simulink model "quad_model_with_pendulum"  (R2016a)
settings: Solver=ode45  StartTime=0.0  StopTime=30  RelTol=1e-3
values from neighbouring files (symbols this model uses):
  disturbance_xy_wind_gain = 0.00    (= 0)    [quad_model_with_pendulum_params.m]
  disturbance_y_delay = 0.5    [quad_model_with_pendulum_params.m]
  gravity = 9.80665    [quad_model_with_pendulum_params.m]
  has_links = 1    [quad_model_with_pendulum_params.m]
  has_sensor = 1    [quad_model_with_pendulum_params.m]
  link_length = 0.25    [quad_model_with_pendulum_params.m]
  link_mass = 0.0075/2    (= 0.00375)    [quad_model_with_pendulum_params.m]
  N = 1    [quaternion.m]
  num_links = 16    [quad_model_with_pendulum_params.m]
  s = ones( size( x ))    [quaternion.m]
  sensor_delay = 0.30    (= 0.3)    [quad_model_with_pendulum_params.m]
  sensor_mass = 0.015    [quad_model_with_pendulum_params.m]
  sensor_sample_time = 0.1    [quad_model_with_pendulum_params.m]
  vehicle_initial_height = -4    [quad_model_with_pendulum_params.m]
  vehicle_mass = 0.550    (= 0.55)    [quad_model_with_pendulum_params.m]
  vehicle_velocity_ascent_limit = -4    [quad_model_with_pendulum_params.m]
  vehicle_velocity_descent_limit = 4.0    (= 4)    [quad_model_with_pendulum_params.m]
  w_ref = 0    [quad_model_with_pendulum_params.m]
  x_Kd = 0.14/n    (= 0.14)    [quad_model_with_pendulum_params.m]
  x_Kp = 0.085/n    (= 0.085)    [quad_model_with_pendulum_params.m]
  x_ref = 1    [quad_model_with_pendulum_params.m]
  Y = [Y(1,:); Y(end,:)]    [quaternion.m]
  y_Kd = 0.14/n    (= 0.14)    [quad_model_with_pendulum_params.m]
  y_Kp = 0.085/n    (= 0.085)    [quad_model_with_pendulum_params.m]
  y_ref = 1    [quad_model_with_pendulum_params.m]
  z_Kd = 1.05    [quad_model_with_pendulum_params.m]
  z_Kp = 0.8    [quad_model_with_pendulum_params.m]
  z_ref = 0.0    (= 0)    [quad_model_with_pendulum_params.m]
undefined symbols (not defined in the file or in its folder): EulerAngles, quaternion, RotateVector, wind_velocity_scale_factor, X, Z
libraries: nesl_utility x21, sm_lib x17, experimental_link_model_x_plus x8, experimental_link_model_x_minus x7, dsparch4 x3, simulink x3, fuzblock x2
settings Model: Creator=jore  LastModifiedBy=jore
settings DataIOCC: LimitDataPoints=on  SaveFormat=Array  OutputTimes=[0:0.3:30]
settings HardwareCC: ProdBitPerPointer=32  ProdLargestAtomicFloat=None  ProdIntDivRoundTo=Undefined  ProdEndianess=Unspecified  ProdWordSize=32  ProdHWDeviceType=32-bit Generic
settings ModelReferenceCC: PropagateSignalLabelsOutOfModel=off
settings ConfigComp: CovModelRefEnable=Off
settings ConfigurationSet: Description=SimMechanics 2G
settings ExplorerConfigSet: InternalSimMechanicsExplorerSettings="<ExplorerConfiguration><canonicalview>aerospace</canonicalview><AnimationSetting><BasePlaybackSpeed>1.0</BasePlaybackSpeed><PlaybackSpeedFactor>1.0</PlaybackSpeedFactor></AnimationSetting><TilePanel><TileInfo><Tiles Columns=\"1\" Count=\"1\" Rows=\"1\"><Column Left=\"2\" Weight=\"1\"/><Column Left=\"883\"/><Row Top=\"2\" Weight=\"1\"/><Row Top=\"2319\"/><Tile Height=\"1\" Width=\"1\" X=\"0\" Y=\"0\"/></Tiles></TileInfo><SceneInfo><SceneViewer><BGColor><R>0.60000002384185791</R><G>0.60000002384185791</G><B>0.60000002384185791</B></BGColor><Camera><DoPerspective>off</DoPerspective><Position><X>0.206725447032578502</X><Y>12.9211399937233526</Y><Z>-2.23169927424554082</Z></Position><Center><X>0.206725447032578502</X><Y>-6.73147066983237341e-07</Y><Z>-2.23169927424554082</Z></Center><Up><X>0</X><Y>0</Y><Z>-1</Z></Up><ViewLimDist>1</ViewLimDist><YLim>10.4733537019934797</YLim><XLim>3.95700365170637491</XLim></Camera></SceneViewer></SceneInfo></TilePanel><MechEditorPanel><Cameras/><GfxPanelCameraMap/></MechEditorPanel></ExplorerConfiguration>"

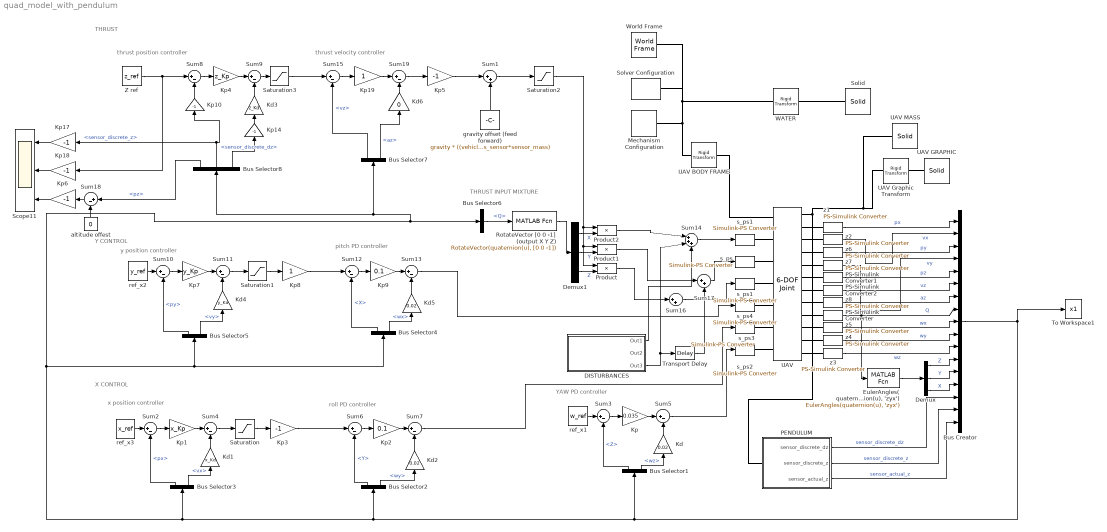
== system quad_model_with_pendulum ==
  note: THRUST INPUT MIXTURE
  note: X CONTROL
  note: THRUST
  note: YAW PD controller
  note: x position controller
  note: roll PD controller
  note: y position controller
  note: pitch PD controller
  note: thrust position controller
  note: thrust velocity controller
  note: Y CONTROL
   s_ps{1..4} (4 alike) : nesl_utility/Simulink-PS Converter  PhysicalDomain=network_engine_domain  SubClassName=ps_input  LeftPortType=input  RightPortType=output  PseudoPeriodic=off  Frequencies=[]  NoiseDistribution=none  NoiseParameters=[]  Unit=1  AffineConversion=off  InputFiltering=off  SimscapeFilterOrder=1  InputFilterTimeConstant=0.001  UdotUserProvided=1
  Bus Creator : BusCreator  Inputs=17
  Bus Selector1 : BusSelector  OutputSignals=Z,wz
  Bus Selector2 : BusSelector  OutputSignals=Y,wy
  Bus Selector3 : BusSelector  OutputSignals=px,vx
  Bus Selector4 : BusSelector  OutputSignals=X,wx
  Bus Selector5 : BusSelector  OutputSignals=py,vy
  Bus Selector6 : BusSelector  OutputSignals=Q
  Bus Selector7 : BusSelector  OutputSignals=vz,az
  Bus Selector8 : BusSelector  OutputSignals=pz,sensor_discrete_z,sensor_discrete_dz
  DISTURBANCES : Subsystem
  Demux : Demux  Outputs=3
  Demux1 : Demux  Outputs=3
  "EulerAngles( quaternion(u), 'zyx')" : MATLABFcn  MATLABFcn=EulerAngles(quaternion(u), 'zyx')  OutputDimensions=3
  Kd : Gain  Gain=0.02
  Kd1 : Gain  Gain=x_Kd
  Kd2 : Gain  Gain=0.02
  Kd3 : Gain  Gain=z_Kd
  Kd4 : Gain  Gain=y_Kd
  Kd5 : Gain  Gain=0.02
  Kd6 : Gain  Gain=0
  Kp : Gain  Gain=0.035
  Kp1 : Gain  Gain=x_Kp
  Kp{3,5..6,10,14,17..18} (7 alike) : Gain  Gain=-1
  Kp19 : Gain
  Kp2 : Gain  Gain=0.1
  Kp4 : Gain  Gain=z_Kp
  Kp7 : Gain  Gain=y_Kp
  Kp8 : Gain
  Kp9 : Gain  Gain=0.1
  Mechanism Configuration : sm_lib/Utilities/Mechanism Configuration  UniformGravity=Constant  GravityVector=[0 0 9.80665]  GravityUnits=m/s^2  LinearizationDelta=0.001
  PENDULUM : Subsystem
  PS-Simulink Converter : nesl_utility/PS-Simulink Converter  PhysicalDomain=network_engine_domain  SubClassName=ps_output  LeftPortType=input  RightPortType=output  PseudoPeriodic=off  Frequencies=[]  Unit=1  AffineConversion=off
  PS-Simulink Converter1 : nesl_utility/PS-Simulink Converter  PhysicalDomain=network_engine_domain  SubClassName=ps_output  LeftPortType=input  RightPortType=output  PseudoPeriodic=off  Frequencies=[]  Unit=1  AffineConversion=off
  PS-Simulink Converter2 : nesl_utility/PS-Simulink Converter  PhysicalDomain=network_engine_domain  SubClassName=ps_output  LeftPortType=input  RightPortType=output  PseudoPeriodic=off  Frequencies=[]  Unit=1  AffineConversion=off
  Product : Product
  Product1 : Product
  Product2 : Product
  RotateVector [0 0 -1] (output X Y Z) : MATLABFcn  MATLABFcn=RotateVector(quaternion(u), [0 0 -1])  OutputDimensions=3
  Saturation : Saturate  UpperLimit=pi/30  LowerLimit=-pi/30
  Saturation1 : Saturate  UpperLimit=pi/30  LowerLimit=-pi/30
  Saturation2 : Saturate  UpperLimit=20  LowerLimit=5.3
  Saturation3 : Saturate  UpperLimit=vehicle_velocity_descent_limit  LowerLimit=vehicle_velocity_ascent_limit
  Scope11 : Scope  NumInputPorts=3
  Solid : sm_lib/Body Elements/Solid  InertiaType=PointMass  Mass=0  MassUnits=kg  CenterOfMass=[0 0 0]  CenterOfMassUnits=m  MomentsOfInertia=[1 1 1]  MomentsOfInertiaUnits=kg*m^2  ProductsOfInertia=[0 0 0]  ProductsOfInertiaUnits=kg*m^2  DensityBased=on  Density=1000  DensityUnits=kg/(m^3)  DoExposeReferenceFrame=on  SerializedFrames=<Frames/>  GraphicType=FromGeometry  MarkerShape=Sphere  MarkerSize=10  MarkerSizeUnits=m  GraphicVisPropType=SimpleVisualProperties  GraphicDiffuseColor=[0.2 0.6 1.0]  GraphicSpecularColor=[0.5 0.5 0.5 1.0]  GraphicAmbientColor=[0.15 0.15 0.15 1.0]  GraphicEmissiveColor=[0.0 0.0 0.0 1.0]  GraphicShininess=75  GraphicOpacity=0.3  GeometryShape=Cylinder  RectangleSize=[1 1]  RectangleSizeUnits=m  BrickDimensions=[1 1 1]  BrickDimensionUnits=m  CylinderRadius=9  CylinderRadiusUnits=m  CylinderLength=4  CylinderLengthUnits=m  SphereRadius=1  SphereRadiusUnits=m  EllipsoidRadii=[1 1 1]  EllipsoidRadiiUnits=m  ExtrusionCrossSection=[1 1; -1 1; -1 -1; 1 -1]  ExtrusionCrossSectionUnits=m  ExtrusionLength=1  ExtrusionLengthUnits=m  PolygonNumSides=3  PolygonOuterRadius=1  PolygonOuterRadiusUnits=m  ExtGeomFileType=STL  ExtGeomFileUnits=m  RevolutionCrossSection=[1 1; 1 -1; 2 -1; 2 1]  RevolutionCrossSectionUnits=m  RevolutionExtent=Full  RevolutionAngle=180  RevolutionAngleUnits=deg
  Solver Configuration : nesl_utility/Solver Configuration  PhysicalDomain=network_engine_domain  SubClassName=solver  LeftPortType=input  RightPortType=generic  Accelerate=off  Tones=[]  Harmonics=[]  SimulateNoise=off  Profile=off  UseLocalSampling=off  EnableSwitchedLinearOptims=on  FrequencyDomain=off  UseCCode=off  RelTol=0.001  AbsTol=1e-06  MinStep=1e-09  ToWorkspace=off  RevertToSquareIcSolve=off  NumHomotopyIterations=100  PhasorMode=off  PhasorModeNumHarmonics=1  OverrideAbsTol=off  DoDC=off  ResidualTolerance=1e-09  UseLocalSolver=off  LocalSolverChoice=NE_BACKWARD_EULER_ADVANCER  LocalSolverSampleTime=0.0001  DoFixedCost=off  MaxNonlinIter=3  MaxModeIter=2  LinearAlgebra=Sparse  DelaysMemoryBudget=1024  AutomaticFiltering=on  FilteringTimeConstant=0.001
  Sum1 : Sum  Inputs=|++
  Sum{2..13,15,18..19} (15 alike) : Sum  Inputs=|+-
  Sum14 : Sum  Inputs=|+++
  Sum16 : Sum  Inputs=|++
  Sum17 : Sum  Inputs=|++
  To Workspace1 : ToWorkspace  VariableName=x1  SaveFormat=Timeseries  SampleTime=-1
  Transport Delay : TransportDelay  DelayTime=disturbance_y_delay
  UAV : sm_lib/Joints/6-DOF Joint  SenseConstraintForce=off  SenseConstraintForceX=off  SenseConstraintForceY=off  SenseConstraintForceZ=off  SenseConstraintTorque=off  SenseConstraintTorqueX=off  SenseConstraintTorqueY=off  SenseConstraintTorqueZ=off  SenseTotalForce=off  SenseTotalForceX=off  SenseTotalForceY=off  SenseTotalForceZ=off  SenseTotalTorque=off  SenseTotalTorqueX=off  SenseTotalTorqueY=off  SenseTotalTorqueZ=off  CompositeWrenchDir=FollowerOnBase  CompositeWrenchFrame=BaseFrame  PxEquilibriumPosition=0  PxEquilibriumPositionUnits=m  PxSpringStiffness=0  PxSpringStiffnessUnits=N/m  PxDampingCoefficient=0  PxDampingCoefficientUnits=N/(m/s)  PxTorqueActuationMode=InputTorque  PxMotionActuationMode=ComputedMotion  PxSensePosition=on  PxSenseVelocity=on  PxSenseAcceleration=off  PxSenseTorqueForce=off  PxPositionTargetSpecify=off  PxPositionTargetPriority=High  PxPositionTargetValue=0  PxPositionTargetValueUnits=m  PxVelocityTargetSpecify=off  PxVelocityTargetPriority=High  PxVelocityTargetValue=0  PxVelocityTargetValueUnits=m/s  PyEquilibriumPosition=0  PyEquilibriumPositionUnits=m  PySpringStiffness=0  PySpringStiffnessUnits=N/m  PyDampingCoefficient=0  PyDampingCoefficientUnits=N/(m/s)  PyTorqueActuationMode=InputTorque  PyMotionActuationMode=ComputedMotion  PySensePosition=on  PySenseVelocity=on  PySenseAcceleration=off  PySenseTorqueForce=off  PyPositionTargetSpecify=off  PyPositionTargetPriority=High  PyPositionTargetValue=0  PyPositionTargetValueUnits=m  PyVelocityTargetSpecify=off  PyVelocityTargetPriority=High  PyVelocityTargetValue=0  PyVelocityTargetValueUnits=m/s  PzEquilibriumPosition=0  PzEquilibriumPositionUnits=m  PzSpringStiffness=0  PzSpringStiffnessUnits=N/m  PzDampingCoefficient=0  PzDampingCoefficientUnits=N/(m/s)  PzTorqueActuationMode=InputTorque  PzMotionActuationMode=ComputedMotion  PzSensePosition=on  PzSenseVelocity=on  PzSenseAcceleration=on  PzSenseTorqueForce=off  PzPositionTargetSpecify=on  PzPositionTargetPriority=High  PzPositionTargetValue=0  PzPositionTargetValueUnits=m  PzVelocityTargetSpecify=off  PzVelocityTargetPriority=High  PzVelocityTargetValue=0  PzVelocityTargetValueUnits=m/s  SphDefPosRotationMethod=None  SphDefPosRotationAngleUnits=deg  SphDefPosRotationStandardAxis=+Z  SphDefPosRotationAngle=0.0  SphDefPosRotationArbitraryAxis=[0 0 1]  SphDefPosFollAlignAxisA=+X  SphDefPosBaseAlignAxisA=+Y  SphDefPosFollAlignAxisB=+Y  SphDefPosBaseAlignAxisB=+Z  SphDefPosRotationSequenceAxes=FollowerAxes  SphDefPosRotationSequence=XYX  SphDefPosRotationSequenceAngles=[0 0 0]  SphDefPosRotationSequenceAnglesUnits=deg  SphDefPosRotationMatrix=[1 0 0; 0 1 0; 0 0 1]  SphEqPosRotationMethod=None  SphEqPosRotationAngleUnits=deg  SphEqPosRotationStandardAxis=+Z  SphEqPosRotationAngle=0.0  SphEqPosRotationArbitraryAxis=[0 0 1]  SphEqPosFollAlignAxisA=+X  SphEqPosBaseAlignAxisA=+Y  SphEqPosFollAlignAxisB=+Y  SphEqPosBaseAlignAxisB=+Z  SphEqPosRotationSequenceAxes=FollowerAxes  SphEqPosRotationSequence=XYX  SphEqPosRotationSequenceAngles=[0 0 0]  SphEqPosRotationSequenceAnglesUnits=deg  SphEqPosRotationMatrix=[1 0 0; 0 1 0; 0 0 1]  SphSpringStiffness=0  SphSpringStiffnessUnits=N*m/deg  SphDampingCoefficient=0  SphDampingCoefficientUnits=N*m/(deg/s)  SphActuateTorqueX=on  SphActuateTorqueY=on  SphActuateTorqueZ=on  SphActuateTorque=off  SphTorqueActuationMode=InputTorque  SphMotionActuationMode=ComputedMotion  SphActuationFrame=BaseFrame  SphSensePosition=on  SphSenseVelocityX=on  SphSenseVelocityY=on  SphSenseVelocityZ=on  SphSenseVelocity=off  SphSenseAccelerationX=off  SphSenseAccelerationY=off  SphSenseAccelerationZ=off  SphSenseAcceleration=off  SphSenseTorqueX=off  SphSenseTorqueY=off  SphSenseTorqueZ=off  SphSenseTorqueForce=off  SphSensingFrame=BaseFrame  SphPositionTargetRotationMethod=None  SphPositionTargetRotationAngleUnits=deg  SphPositionTargetRotationStandardAxis=+Z  SphPositionTargetRotationAngle=0.0  SphPositionTargetRotationArbitraryAxis=[0 0 1]  SphPositionTargetFollAlignAxisA=+X  SphPositionTargetBaseAlignAxisA=+Y  SphPositionTargetFollAlignAxisB=+Y  SphPositionTargetBaseAlignAxisB=+Z  SphPositionTargetRotationSequenceAxes=FollowerAxes  SphPositionTargetRotationSequence=XYX  SphPositionTargetRotationSequenceAngles=[0 0 0]  SphPositionTargetRotationSequenceAnglesUnits=deg  SphPositionTargetRotationMatrix=[1 0 0; 0 1 0; 0 0 1]  SphPositionTargetSpecify=off  SphPositionTargetPriority=High  SphVelocityTargetValue=[0 0 0]  SphVelocityTargetValueUnits=deg/s  SphVelocityTargetSpecify=off  SphVelocityTargetPriority=High  SphVelocityTargetInFollowerFrame=on
  UAV BODY FRAME : sm_lib/Frames and Transforms/Rigid Transform  TranslationMethod=Cartesian  TranslationLengthUnit=m  TranslationStandardAxis=-Z  TranslationStandardOffset=num_links*link_length  TranslationCartesianOffset="[0 0  vehicle_initial_height]"  TranslationROffset=0  TranslationROffsetUnits=m  TranslationZOffset=0  TranslationZOffsetUnits=m  TranslationThetaOffset=0  TranslationThetaOffsetUnits=deg  RotationMethod=None  RotationAngleUnits=deg  RotationStandardAxis=+X  RotationAngle=90  RotationArbitraryAxis=[0 1 1]  FollAlignAxisA=+X  BaseAlignAxisA=+Y  FollAlignAxisB=+Y  BaseAlignAxisB=+Z  RotationSequenceAxes=FollowerAxes  RotationSequence=XYX  RotationSequenceAngles=[0 0 0]  RotationSequenceAnglesUnits=deg  RotationMatrix=[0 0 1; -1 0 0; 0 -1 0]
  UAV GRAPHIC : sm_lib/Body Elements/Solid  InertiaType=PointMass  Mass=0  MassUnits=kg  CenterOfMass=[0 0 0]  CenterOfMassUnits=m  MomentsOfInertia=[1 1 1]  MomentsOfInertiaUnits=kg*m^2  ProductsOfInertia=[0 0 0]  ProductsOfInertiaUnits=kg*m^2  DensityBased=off  Density=1000  DensityUnits=kg/(m^3)  DoExposeReferenceFrame=on  SerializedFrames=<Frames/>  GraphicType=FromGeometry  MarkerShape=Sphere  MarkerSize=10  MarkerSizeUnits=m  GraphicVisPropType=SimpleVisualProperties  GraphicDiffuseColor=[0.3 0.3 0.3]  GraphicSpecularColor=[0.5 0.5 0.5 1.0]  GraphicAmbientColor=[0.15 0.15 0.15 1.0]  GraphicEmissiveColor=[0.0 0.0 0.0 1.0]  GraphicShininess=75  GraphicOpacity=1.0  GeometryShape=FromFile  RectangleSize=[1 1]  RectangleSizeUnits=m  BrickDimensions=[1 1 1]  BrickDimensionUnits=m  CylinderRadius=1  CylinderRadiusUnits=m  CylinderLength=1  CylinderLengthUnits=m  SphereRadius=1  SphereRadiusUnits=m  EllipsoidRadii=[1 1 1]  EllipsoidRadiiUnits=m  ExtrusionCrossSection=[1 1; -1 1; -1 -1; 1 -1]  ExtrusionCrossSectionUnits=m  ExtrusionLength=1  ExtrusionLengthUnits=m  PolygonNumSides=3  PolygonOuterRadius=1  PolygonOuterRadiusUnits=m  ExtGeomFileType=STL  ExtGeomFileName=Top Level Hummingbird Part.STL  ExtGeomFileUnits=mm  RevolutionCrossSection=[1 1; 1 -1; 2 -1; 2 1]  RevolutionCrossSectionUnits=m  RevolutionExtent=Full  RevolutionAngle=180  RevolutionAngleUnits=deg
  UAV Graphic Transform : sm_lib/Frames and Transforms/Rigid Transform  TranslationMethod=Cartesian  TranslationLengthUnit=m  TranslationStandardAxis=+Z  TranslationStandardOffset=0  TranslationCartesianOffset=[-0.275 0.238 0.02]  TranslationROffset=0  TranslationROffsetUnits=m  TranslationZOffset=0  TranslationZOffsetUnits=m  TranslationThetaOffset=0  TranslationThetaOffsetUnits=deg  RotationMethod=RotationMatrix  RotationAngleUnits=deg  RotationStandardAxis=+X  RotationAngle=90  RotationArbitraryAxis=[0 1 1]  FollAlignAxisA=+X  BaseAlignAxisA=+Y  FollAlignAxisB=+Y  BaseAlignAxisB=+Z  RotationSequenceAxes=FollowerAxes  RotationSequence=XYX  RotationSequenceAngles=[0 0 0]  RotationSequenceAnglesUnits=deg  RotationMatrix=[0 0 1; -1 0 0; 0 -1 0]
  UAV MASS : sm_lib/Body Elements/Solid  InertiaType=CalculateFromGeometry  Mass=vehicle_mass  MassUnits=kg  CenterOfMass=[0 0 0]  CenterOfMassUnits=m  MomentsOfInertia=[1 1 1]  MomentsOfInertiaUnits=kg*m^2  ProductsOfInertia=[0 0 0]  ProductsOfInertiaUnits=kg*m^2  DensityBased=off  Density=1  DensityUnits=kg/(m^3)  DoExposeReferenceFrame=on  SerializedFrames=<Frames/>  GraphicType=None  MarkerShape=Sphere  MarkerSize=10  MarkerSizeUnits=m  GraphicVisPropType=SimpleVisualProperties  GraphicDiffuseColor=[1.0 1.0 0.2]  GraphicSpecularColor=[0.5 0.5 0.5 1.0]  GraphicAmbientColor=[0.15 0.15 0.15 1.0]  GraphicEmissiveColor=[0.0 0.0 0.0 1.0]  GraphicShininess=75  GraphicOpacity=0.1  GeometryShape=Sphere  RectangleSize=[1 1]  RectangleSizeUnits=m  BrickDimensions=[1 1 1]  BrickDimensionUnits=m  CylinderRadius=1  CylinderRadiusUnits=m  CylinderLength=1  CylinderLengthUnits=m  SphereRadius=0.1  SphereRadiusUnits=m  EllipsoidRadii=[1 1 1]  EllipsoidRadiiUnits=m  ExtrusionCrossSection=[1 1; -1 1; -1 -1; 1 -1]  ExtrusionCrossSectionUnits=m  ExtrusionLength=1  ExtrusionLengthUnits=m  PolygonNumSides=3  PolygonOuterRadius=1  PolygonOuterRadiusUnits=m  ExtGeomFileType=STL  ExtGeomFileUnits=m  RevolutionCrossSection=[1 1; 1 -1; 2 -1; 2 1]  RevolutionCrossSectionUnits=m  RevolutionExtent=Full  RevolutionAngle=180  RevolutionAngleUnits=deg
  WATER : sm_lib/Frames and Transforms/Rigid Transform  TranslationMethod=StandardAxis  TranslationLengthUnit=m  TranslationStandardAxis=+Z  TranslationStandardOffset=2  TranslationCartesianOffset=[-0.275 0.238 0.02]  TranslationROffset=0  TranslationROffsetUnits=m  TranslationZOffset=0  TranslationZOffsetUnits=m  TranslationThetaOffset=0  TranslationThetaOffsetUnits=deg  RotationMethod=None  RotationAngleUnits=deg  RotationStandardAxis=+X  RotationAngle=90  RotationArbitraryAxis=[0 1 1]  FollAlignAxisA=+X  BaseAlignAxisA=+Y  FollAlignAxisB=+Y  BaseAlignAxisB=+Z  RotationSequenceAxes=FollowerAxes  RotationSequence=XYX  RotationSequenceAngles=[0 0 0]  RotationSequenceAnglesUnits=deg  RotationMatrix=[0 0 1; -1 0 0; 0 -1 0]
  World Frame : sm_lib/Frames and Transforms/World Frame
  "Z ref " : Constant  Value=z_ref
  altitude offest : Constant  Value=0
  gravity offset (feed forward) : Constant  Value=gravity * ((vehicle_mass) + has_links*(num_links * link_mass) + has_sensor*sensor_mass)
  ref_x1 : Constant  Value=w_ref
  ref_x2 : Constant  Value=y_ref
  ref_x3 : Constant  Value=x_ref
  s_ps : nesl_utility/Simulink-PS Converter  PhysicalDomain=network_engine_domain  SubClassName=ps_input  LeftPortType=input  RightPortType=output  PseudoPeriodic=off  Frequencies=[]  NoiseDistribution=none  NoiseParameters=[]  Unit=1  AffineConversion=off  InputFiltering=off  SimscapeFilterOrder=1  InputFilterTimeConstant=0.001  UdotUserProvided=1
  s_ps1 : nesl_utility/Simulink-PS Converter  PhysicalDomain=network_engine_domain  SubClassName=ps_input  LeftPortType=input  RightPortType=output  PseudoPeriodic=off  Frequencies=[]  NoiseDistribution=none  NoiseParameters=[]  Unit=1  AffineConversion=off  InputFiltering=off  SimscapeFilterOrder=1  InputFilterTimeConstant=0.001  UdotUserProvided=1
  z{1..8} (8 alike) : nesl_utility/PS-Simulink Converter  PhysicalDomain=network_engine_domain  SubClassName=ps_output  LeftPortType=input  RightPortType=output  PseudoPeriodic=off  Frequencies=[]  Unit=1  AffineConversion=off
  wires:
  PS-Simulink Converter/1 -> Bus Creator/8, "EulerAngles( quaternion(u), 'zyx')"/1  "Q"
  "EulerAngles( quaternion(u), 'zyx')"/1 -> Demux/1
  Demux/1 -> Bus Creator/12  "Z"
  Kd/1 -> Sum5/2
  z3/1 -> Bus Creator/11  "wz"
  Sum3/1 -> Kp/1
  Kp/1 -> Sum5/1
  ref_x1/1 -> Sum3/1
  RotateVector [0 0 -1] (output X Y Z)/1 -> Demux1/1
  Demux1/3 -> Product/2  "Z"
  gravity offset (feed forward)/1 -> Sum1/2
  Demux1/1 -> Product2/2  "X"
  Demux1/2 -> Product1/2  "Y"
  Sum5/1 -> " s_ps2"/1
  Sum2/1 -> Kp1/1
  Kp1/1 -> Sum4/1
  ref_x3/1 -> Sum2/1
  z1/1 -> Bus Creator/1  "px"
  Product2/1 -> Sum14/1
  Product/1 -> Sum16/1
  Kd2/1 -> Sum7/2
  Sum6/1 -> Kp2/1
  Kp2/1 -> Sum7/1
  Demux/2 -> Bus Creator/13  "Y"
  z4/1 -> Bus Creator/10  "wy"
  Sum4/1 -> Saturation/1
  Sum7/1 -> " s_ps3"/1
  Saturation/1 -> Kp3/1
  Kp3/1 -> Sum6/1
  Kd1/1 -> Sum4/2
  z2/1 -> Bus Creator/2  "vx"
  Sum8/1 -> Kp4/1
  Kp4/1 -> Sum9/1
  "Z ref "/1 -> Kp18/1, Sum8/1
  PS-Simulink Converter1/1 -> Bus Creator/5  "pz"
  PS-Simulink Converter2/1 -> Bus Creator/6  "vz"
  Kp5/1 -> Sum1/1
  Kd3/1 -> Sum9/2
  Kp6/1 -> Scope11/3
  Sum10/1 -> Kp7/1
  Kp7/1 -> Sum11/1
  ref_x2/1 -> Sum10/1
  Sum11/1 -> Saturation1/1
  Saturation1/1 -> Kp8/1
  Kd4/1 -> Sum11/2
  Kd5/1 -> Sum13/2
  Sum12/1 -> Kp9/1
  Kp9/1 -> Sum13/1
  Kp8/1 -> Sum12/1
  Demux/3 -> Bus Creator/14  "X"
  z5/1 -> Bus Creator/9  "wx"
  z6/1 -> Bus Creator/3  "py"
  z7/1 -> Bus Creator/4  "vy"
  Sum13/1 -> " s_ps4"/1
  Sum1/1 -> Saturation2/1
  Saturation2/1 -> Product2/1, Product1/1, Product/1
  Sum14/1 -> s_ps1/1
  Product1/1 -> Sum17/1
  Kp14/1 -> Kd3/1
  PENDULUM/1(sensor_discrete_dz) -> Bus Creator/15  "sensor_discrete_dz"
  PENDULUM/2(sensor_discrete_z) -> Bus Creator/16  "sensor_discrete_z"
  Sum16/1 -> " s_ps1"/1
  Kp17/1 -> Scope11/1
  Sum17/1 -> s_ps/1
  Transport Delay/1 -> Sum17/2
  altitude offest/1 -> Sum18/2
  Sum18/1 -> Kp6/1
  Kp18/1 -> Scope11/2
  Kd6/1 -> Sum19/2
  Sum9/1 -> Saturation3/1
  Sum15/1 -> Kp19/1
  Kp19/1 -> Sum19/1
  Saturation3/1 -> Sum15/1
  Sum19/1 -> Kp5/1
  z8/1 -> Bus Creator/7  "az"
  Bus Creator/1 -> To Workspace1/1, Bus Selector3/1, Bus Selector4/1, Bus Selector5/1, Bus Selector6/1, Bus Selector8/1, Bus Selector7/1, Bus Selector2/1, Bus Selector1/1
  Bus Selector1/2 -> Kd/1  "<wz>"
  Bus Selector1/1 -> Sum3/2  "<Z>"
  Bus Selector2/2 -> Kd2/1  "<wy>"
  Bus Selector2/1 -> Sum6/2  "<Y>"
  Bus Selector3/2 -> Kd1/1  "<vx>"
  Bus Selector3/1 -> Sum2/2  "<px>"
  Bus Selector4/2 -> Kd5/1  "<wx>"
  Bus Selector4/1 -> Sum12/2  "<X>"
  Bus Selector5/2 -> Kd4/1  "<vy>"
  Bus Selector5/1 -> Sum10/2  "<py>"
  Bus Selector6/1 -> RotateVector [0 0 -1] (output X Y Z)/1  "<Q>"
  Bus Selector7/2 -> Kd6/1  "<az>"
  Bus Selector7/1 -> Sum15/2  "<vz>"
  DISTURBANCES/3(Out3) -> Sum14/2, Transport Delay/1
  DISTURBANCES/1(Out1) -> Sum14/3
  Kp10/1 -> Sum8/2
  Bus Selector8/3 -> Kp14/1  "<sensor_discrete_dz>"
  Bus Selector8/2 -> Kp10/1, Kp17/1  "<sensor_discrete_z>"
  Bus Selector8/1 -> Sum18/1  "<pz>"
  PENDULUM/3(sensor_actual_z) -> Bus Creator/17  "sensor_actual_z"
  connections:
  UAV GRAPHIC/RConn1 -- UAV Graphic Transform/RConn1
  " s_ps1"/RConn1 -- UAV/LConn4
  PS-Simulink Converter/LConn1 -- UAV/RConn9
  " s_ps2"/RConn1 -- UAV/LConn7
  s_ps/RConn1 -- UAV/LConn3
  s_ps1/RConn1 -- UAV/LConn2
  " s_ps3"/RConn1 -- UAV/LConn6
  " s_ps4"/RConn1 -- UAV/LConn5
  UAV/RConn12 -- z3/LConn1
  z1/LConn1 -- UAV/RConn2
  z2/LConn1 -- UAV/RConn3
  z4/LConn1 -- UAV/RConn11
  PS-Simulink Converter1/LConn1 -- UAV/RConn6
  UAV/RConn7 -- PS-Simulink Converter2/LConn1
  UAV/RConn10 -- z5/LConn1
  z6/LConn1 -- UAV/RConn4
  z7/LConn1 -- UAV/RConn5
  UAV BODY FRAME/RConn1 -- UAV/LConn1
  UAV MASS/RConn1 -- UAV Graphic Transform/LConn1 -- PENDULUM/LConn1 -- UAV/RConn1
  Mechanism Configuration/RConn1 -- WATER/LConn1 -- World Frame/RConn1 -- Solver Configuration/RConn1 -- UAV BODY FRAME/LConn1
  z8/LConn1 -- UAV/RConn8
  WATER/RConn1 -- Solid/RConn1

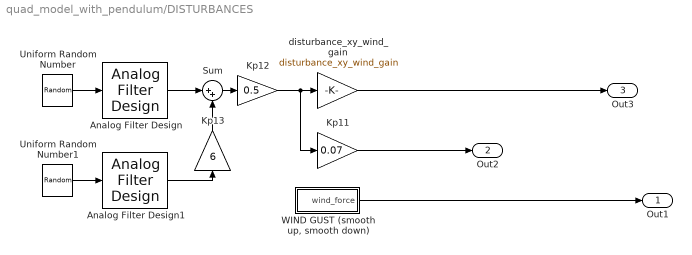
== system quad_model_with_pendulum/DISTURBANCES ==
  Analog Filter Design : dsparch4/Analog Filter Design  method=Butterworth  filttype=Lowpass  N=8  Wlo=30  Whi=80  Rp=2  Rs=40
  Analog Filter Design1 : dsparch4/Analog Filter Design  method=Butterworth  filttype=Lowpass  N=8  Wlo=30  Whi=80  Rp=2  Rs=40
  Kp11 : Gain  Gain=0.07
  Kp12 : Gain  Gain=0.5
  Kp13 : Gain  Gain=6
  Sum : Sum  Inputs=|++
  Uniform Random Number : UniformRandomNumber  SampleTime=0.5
  Uniform Random Number1 : UniformRandomNumber  SampleTime=4
  "WIND GUST (smooth up, smooth down) " : Subsystem
  disturbance_xy_wind_gain : Gain  Gain=disturbance_xy_wind_gain
  Out1 : Outport
  Out2 : Outport  Port=2
  Out3 : Outport  Port=3
  wires:
  Uniform Random Number/1 -> Analog Filter Design/1
  Kp12/1 -> Kp11/1, disturbance_xy_wind_gain/1
  disturbance_xy_wind_gain/1 -> Out3/1
  Analog Filter Design/1 -> Sum/1
  Uniform Random Number1/1 -> Analog Filter Design1/1
  Analog Filter Design1/1 -> Kp13/1
  Sum/1 -> Kp12/1
  Kp13/1 -> Sum/2
  Kp11/1 -> Out2/1
  "WIND GUST (smooth up, smooth down) "/1(wind_force) -> Out1/1

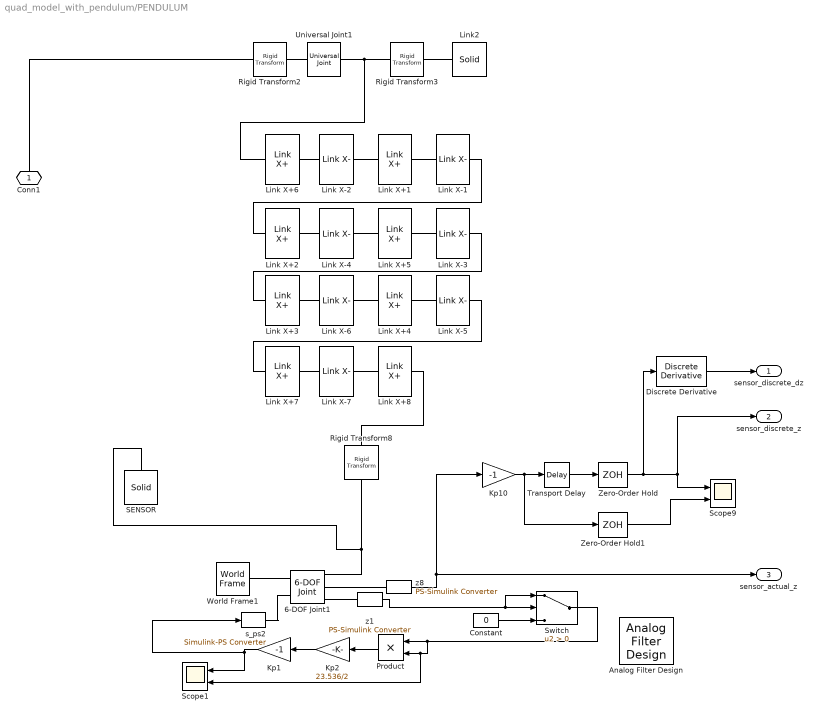
== system quad_model_with_pendulum/PENDULUM ==
  " s_ps2" : nesl_utility/Simulink-PS Converter  PhysicalDomain=network_engine_domain  SubClassName=ps_input  LeftPortType=input  RightPortType=output  PseudoPeriodic=off  Frequencies=[]  NoiseDistribution=none  NoiseParameters=[]  Unit=1  AffineConversion=off  InputFiltering=off  SimscapeFilterOrder=1  InputFilterTimeConstant=0.001  UdotUserProvided=1
  6-DOF Joint1 : sm_lib/Joints/6-DOF Joint  SenseConstraintForce=off  SenseConstraintForceX=off  SenseConstraintForceY=off  SenseConstraintForceZ=off  SenseConstraintTorque=off  SenseConstraintTorqueX=off  SenseConstraintTorqueY=off  SenseConstraintTorqueZ=off  SenseTotalForce=off  SenseTotalForceX=off  SenseTotalForceY=off  SenseTotalForceZ=off  SenseTotalTorque=off  SenseTotalTorqueX=off  SenseTotalTorqueY=off  SenseTotalTorqueZ=off  CompositeWrenchDir=FollowerOnBase  CompositeWrenchFrame=BaseFrame  PxEquilibriumPosition=0  PxEquilibriumPositionUnits=m  PxSpringStiffness=0  PxSpringStiffnessUnits=N/m  PxDampingCoefficient=pendulum_sensor_damping_xy  PxDampingCoefficientUnits=N/(m/s)  PxTorqueActuationMode=NoTorque  PxMotionActuationMode=ComputedMotion  PxSensePosition=off  PxSenseVelocity=off  PxSenseAcceleration=off  PxSenseTorqueForce=off  PxPositionTargetSpecify=off  PxPositionTargetPriority=High  PxPositionTargetValue=0  PxPositionTargetValueUnits=m  PxVelocityTargetSpecify=off  PxVelocityTargetPriority=High  PxVelocityTargetValue=0  PxVelocityTargetValueUnits=m/s  PyEquilibriumPosition=0  PyEquilibriumPositionUnits=m  PySpringStiffness=0  PySpringStiffnessUnits=N/m  PyDampingCoefficient=pendulum_sensor_damping_xy  PyDampingCoefficientUnits=N/(m/s)  PyTorqueActuationMode=NoTorque  PyMotionActuationMode=ComputedMotion  PySensePosition=off  PySenseVelocity=off  PySenseAcceleration=off  PySenseTorqueForce=off  PyPositionTargetSpecify=off  PyPositionTargetPriority=High  PyPositionTargetValue=0  PyPositionTargetValueUnits=m  PyVelocityTargetSpecify=off  PyVelocityTargetPriority=High  PyVelocityTargetValue=0  PyVelocityTargetValueUnits=m/s  PzEquilibriumPosition=0  PzEquilibriumPositionUnits=m  PzSpringStiffness=0  PzSpringStiffnessUnits=N/m  PzDampingCoefficient=0  PzDampingCoefficientUnits=N/(m/s)  PzTorqueActuationMode=InputTorque  PzMotionActuationMode=ComputedMotion  PzSensePosition=on  PzSenseVelocity=on  PzSenseAcceleration=off  PzSenseTorqueForce=off  PzPositionTargetSpecify=off  PzPositionTargetPriority=High  PzPositionTargetValue=0  PzPositionTargetValueUnits=m  PzVelocityTargetSpecify=off  PzVelocityTargetPriority=High  PzVelocityTargetValue=0  PzVelocityTargetValueUnits=m/s  SphDefPosRotationMethod=None  SphDefPosRotationAngleUnits=deg  SphDefPosRotationStandardAxis=+Z  SphDefPosRotationAngle=0.0  SphDefPosRotationArbitraryAxis=[0 0 1]  SphDefPosFollAlignAxisA=+X  SphDefPosBaseAlignAxisA=+Y  SphDefPosFollAlignAxisB=+Y  SphDefPosBaseAlignAxisB=+Z  SphDefPosRotationSequenceAxes=FollowerAxes  SphDefPosRotationSequence=XYX  SphDefPosRotationSequenceAngles=[0 0 0]  SphDefPosRotationSequenceAnglesUnits=deg  SphDefPosRotationMatrix=[1 0 0; 0 1 0; 0 0 1]  SphEqPosRotationMethod=None  SphEqPosRotationAngleUnits=deg  SphEqPosRotationStandardAxis=+Z  SphEqPosRotationAngle=0.0  SphEqPosRotationArbitraryAxis=[0 0 1]  SphEqPosFollAlignAxisA=+X  SphEqPosBaseAlignAxisA=+Y  SphEqPosFollAlignAxisB=+Y  SphEqPosBaseAlignAxisB=+Z  SphEqPosRotationSequenceAxes=FollowerAxes  SphEqPosRotationSequence=XYX  SphEqPosRotationSequenceAngles=[0 0 0]  SphEqPosRotationSequenceAnglesUnits=deg  SphEqPosRotationMatrix=[1 0 0; 0 1 0; 0 0 1]  SphSpringStiffness=0  SphSpringStiffnessUnits=N*m/deg  SphDampingCoefficient=0  SphDampingCoefficientUnits=N*m/(deg/s)  SphActuateTorqueX=off  SphActuateTorqueY=off  SphActuateTorqueZ=off  SphActuateTorque=off  SphTorqueActuationMode=NoTorque  SphMotionActuationMode=ComputedMotion  SphActuationFrame=BaseFrame  SphSensePosition=off  SphSenseVelocityX=off  SphSenseVelocityY=off  SphSenseVelocityZ=off  SphSenseVelocity=off  SphSenseAccelerationX=off  SphSenseAccelerationY=off  SphSenseAccelerationZ=off  SphSenseAcceleration=off  SphSenseTorqueX=off  SphSenseTorqueY=off  SphSenseTorqueZ=off  SphSenseTorqueForce=off  SphSensingFrame=BaseFrame  SphPositionTargetRotationMethod=None  SphPositionTargetRotationAngleUnits=deg  SphPositionTargetRotationStandardAxis=+Z  SphPositionTargetRotationAngle=0.0  SphPositionTargetRotationArbitraryAxis=[0 0 1]  SphPositionTargetFollAlignAxisA=+X  SphPositionTargetBaseAlignAxisA=+Y  SphPositionTargetFollAlignAxisB=+Y  SphPositionTargetBaseAlignAxisB=+Z  SphPositionTargetRotationSequenceAxes=FollowerAxes  SphPositionTargetRotationSequence=XYX  SphPositionTargetRotationSequenceAngles=[0 0 0]  SphPositionTargetRotationSequenceAnglesUnits=deg  SphPositionTargetRotationMatrix=[1 0 0; 0 1 0; 0 0 1]  SphPositionTargetSpecify=off  SphPositionTargetPriority=High  SphVelocityTargetValue=[0 0 0]  SphVelocityTargetValueUnits=deg/s  SphVelocityTargetSpecify=off  SphVelocityTargetPriority=High  SphVelocityTargetInFollowerFrame=on
  Analog Filter Design : dsparch4/Analog Filter Design  method=Butterworth  filttype=Lowpass  N=8  Wlo=30  Whi=80  Rp=2  Rs=40
  Constant : Constant  Value=0
  Discrete Derivative : simulink/Discrete/Discrete Derivative  gainval=1.0  ICPrevScaledInput=0.0  InputProcessing=Inherited  OutMin=[]  OutMax=[]  OutDataType=fixdt(1, 16)  OutScaling=2^-10  DoSatur=off
  Kp1 : Gain  Gain=-1
  Kp10 : Gain  Gain=-1
  Kp2 : Gain  Gain=23.536/2
  Link X+{1..8} (8 alike) : experimental_link_model_x_plus/Link X+
  Link X-{1..7} (7 alike) : experimental_link_model_x_minus/Link X-
  Link2 : sm_lib/Body Elements/Solid  InertiaType=PointMass  Mass=link_mass  MassUnits=kg  CenterOfMass=[0 0 0]  CenterOfMassUnits=m  MomentsOfInertia=[1 1 1]  MomentsOfInertiaUnits=kg*m^2  ProductsOfInertia=[0 0 0]  ProductsOfInertiaUnits=kg*m^2  DensityBased=on  Density=1000  DensityUnits=kg/(m^3)  DoExposeReferenceFrame=on  SerializedFrames=<Frames/>  GraphicType=FromGeometry  MarkerShape=Sphere  MarkerSize=10  MarkerSizeUnits=m  GraphicVisPropType=SimpleVisualProperties  GraphicDiffuseColor=[0.9 0.5 0.5]  GraphicSpecularColor=[0.5 0.5 0.5 1.0]  GraphicAmbientColor=[0.15 0.15 0.15 1.0]  GraphicEmissiveColor=[0.0 0.0 0.0 1.0]  GraphicShininess=75  GraphicOpacity=1.0  GeometryShape=Cylinder  RectangleSize=[1 1]  RectangleSizeUnits=m  BrickDimensions=[1 1 1]  BrickDimensionUnits=m  CylinderRadius=0.0025  CylinderRadiusUnits=m  CylinderLength=0.5  CylinderLengthUnits=m  SphereRadius=1  SphereRadiusUnits=m  EllipsoidRadii=[1 1 1]  EllipsoidRadiiUnits=m  ExtrusionCrossSection=[1 1; -1 1; -1 -1; 1 -1]  ExtrusionCrossSectionUnits=m  ExtrusionLength=1  ExtrusionLengthUnits=m  PolygonNumSides=3  PolygonOuterRadius=1  PolygonOuterRadiusUnits=m  ExtGeomFileType=STL  ExtGeomFileUnits=m  RevolutionCrossSection=[1 1; 1 -1; 2 -1; 2 1]  RevolutionCrossSectionUnits=m  RevolutionExtent=Full  RevolutionAngle=180  RevolutionAngleUnits=deg
  Product : Product
  Rigid Transform2 : sm_lib/Frames and Transforms/Rigid Transform  TranslationMethod=StandardAxis  TranslationLengthUnit=m  TranslationStandardAxis=+Z  TranslationStandardOffset=0.0  TranslationCartesianOffset=[0 0 0]  TranslationROffset=0  TranslationROffsetUnits=m  TranslationZOffset=0  TranslationZOffsetUnits=m  TranslationThetaOffset=0  TranslationThetaOffsetUnits=deg  RotationMethod=StandardAxis  RotationAngleUnits=deg  RotationStandardAxis=-X  RotationAngle=3  RotationArbitraryAxis=[0 0 1]  FollAlignAxisA=+X  BaseAlignAxisA=+Y  FollAlignAxisB=+Y  BaseAlignAxisB=+Z  RotationSequenceAxes=FollowerAxes  RotationSequence=XYX  RotationSequenceAngles=[0 0 0]  RotationSequenceAnglesUnits=deg  RotationMatrix=[1 0 0; 0 1 0; 0 0 1]
  Rigid Transform3 : sm_lib/Frames and Transforms/Rigid Transform  TranslationMethod=StandardAxis  TranslationLengthUnit=m  TranslationStandardAxis=+Z  TranslationStandardOffset=link_length  TranslationCartesianOffset=[0 0 0]  TranslationROffset=0  TranslationROffsetUnits=m  TranslationZOffset=0  TranslationZOffsetUnits=m  TranslationThetaOffset=0  TranslationThetaOffsetUnits=deg  RotationMethod=None  RotationAngleUnits=deg  RotationStandardAxis=+Z  RotationAngle=0.0  RotationArbitraryAxis=[0 0 1]  FollAlignAxisA=+X  BaseAlignAxisA=+Y  FollAlignAxisB=+Y  BaseAlignAxisB=+Z  RotationSequenceAxes=FollowerAxes  RotationSequence=XYX  RotationSequenceAngles=[0 0 0]  RotationSequenceAnglesUnits=deg  RotationMatrix=[1 0 0; 0 1 0; 0 0 1]
  Rigid Transform8 : sm_lib/Frames and Transforms/Rigid Transform  TranslationMethod=StandardAxis  TranslationLengthUnit=m  TranslationStandardAxis=+Z  TranslationStandardOffset=link_length  TranslationCartesianOffset=[0 0 0]  TranslationROffset=0  TranslationROffsetUnits=m  TranslationZOffset=0  TranslationZOffsetUnits=m  TranslationThetaOffset=0  TranslationThetaOffsetUnits=deg  RotationMethod=StandardAxis  RotationAngleUnits=deg  RotationStandardAxis=+Z  RotationAngle=0.0  RotationArbitraryAxis=[0 0 1]  FollAlignAxisA=+X  BaseAlignAxisA=+Y  FollAlignAxisB=+Y  BaseAlignAxisB=+Z  RotationSequenceAxes=FollowerAxes  RotationSequence=XYX  RotationSequenceAngles=[0 0 0]  RotationSequenceAnglesUnits=deg  RotationMatrix=[1 0 0; 0 1 0; 0 0 1]
  SENSOR : sm_lib/Body Elements/Solid  InertiaType=PointMass  Mass=sensor_mass  MassUnits=kg  CenterOfMass=[0 0 0]  CenterOfMassUnits=m  MomentsOfInertia=[1 1 1]  MomentsOfInertiaUnits=kg*m^2  ProductsOfInertia=[0 0 0]  ProductsOfInertiaUnits=kg*m^2  DensityBased=on  Density=1000  DensityUnits=kg/(m^3)  DoExposeReferenceFrame=on  SerializedFrames=<Frames/>  GraphicType=FromGeometry  MarkerShape=Sphere  MarkerSize=10  MarkerSizeUnits=m  GraphicVisPropType=SimpleVisualProperties  GraphicDiffuseColor=[1 0 0 ]  GraphicSpecularColor=[0.5 0.5 0.5 1.0]  GraphicAmbientColor=[0.15 0.15 0.15 1.0]  GraphicEmissiveColor=[0.0 0.0 0.0 1.0]  GraphicShininess=75  GraphicOpacity=0.6  GeometryShape=Sphere  RectangleSize=[1 1]  RectangleSizeUnits=m  BrickDimensions=[1 1 1]  BrickDimensionUnits=m  CylinderRadius=1  CylinderRadiusUnits=m  CylinderLength=1  CylinderLengthUnits=m  SphereRadius=0.02  SphereRadiusUnits=m  EllipsoidRadii=[1 1 1]  EllipsoidRadiiUnits=m  ExtrusionCrossSection=[1 1; -1 1; -1 -1; 1 -1]  ExtrusionCrossSectionUnits=m  ExtrusionLength=1  ExtrusionLengthUnits=m  PolygonNumSides=3  PolygonOuterRadius=1  PolygonOuterRadiusUnits=m  ExtGeomFileType=STL  ExtGeomFileUnits=m  RevolutionCrossSection=[1 1; 1 -1; 2 -1; 2 1]  RevolutionCrossSectionUnits=m  RevolutionExtent=Full  RevolutionAngle=180  RevolutionAngleUnits=deg
  Scope1 : Scope  NumInputPorts=2
  Scope9 : Scope  NumInputPorts=2
  Switch : Switch  Criteria=u2 > Threshold
  Transport Delay : TransportDelay  DelayTime=sensor_delay
  Universal Joint1 : sm_lib/Joints/Universal Joint  SenseConstraintForce=off  SenseConstraintForceX=off  SenseConstraintForceY=off  SenseConstraintForceZ=off  SenseConstraintTorque=off  SenseConstraintTorqueX=off  SenseConstraintTorqueY=off  SenseConstraintTorqueZ=off  SenseTotalForce=off  SenseTotalForceX=off  SenseTotalForceY=off  SenseTotalForceZ=off  SenseTotalTorque=off  SenseTotalTorqueX=off  SenseTotalTorqueY=off  SenseTotalTorqueZ=off  CompositeWrenchDir=FollowerOnBase  CompositeWrenchFrame=BaseFrame  RxEquilibriumPosition=0  RxEquilibriumPositionUnits=deg  RxSpringStiffness=0  RxSpringStiffnessUnits=N*m/deg  RxDampingCoefficient=pendulum_joint_damping  RxDampingCoefficientUnits=N*m/(deg/s)  RxTorqueActuationMode=NoTorque  RxMotionActuationMode=ComputedMotion  RxSensePosition=off  RxSenseVelocity=off  RxSenseAcceleration=off  RxSenseTorqueForce=off  RxPositionTargetSpecify=off  RxPositionTargetPriority=High  RxPositionTargetValue=0  RxPositionTargetValueUnits=deg  RxVelocityTargetSpecify=off  RxVelocityTargetPriority=High  RxVelocityTargetValue=0  RxVelocityTargetValueUnits=deg/s  RyEquilibriumPosition=0  RyEquilibriumPositionUnits=deg  RySpringStiffness=0  RySpringStiffnessUnits=N*m/deg  RyDampingCoefficient=pendulum_joint_damping  RyDampingCoefficientUnits=N*m/(deg/s)  RyTorqueActuationMode=NoTorque  RyMotionActuationMode=ComputedMotion  RySensePosition=off  RySenseVelocity=off  RySenseAcceleration=off  RySenseTorqueForce=off  RyPositionTargetSpecify=off  RyPositionTargetPriority=High  RyPositionTargetValue=0  RyPositionTargetValueUnits=deg  RyVelocityTargetSpecify=off  RyVelocityTargetPriority=High  RyVelocityTargetValue=0  RyVelocityTargetValueUnits=deg/s
  World Frame1 : sm_lib/Frames and Transforms/World Frame
  Zero-Order Hold : ZeroOrderHold  SampleTime=sensor_sample_time
  Zero-Order Hold1 : ZeroOrderHold  SampleTime=sensor_sample_time
  z1 : nesl_utility/PS-Simulink Converter  PhysicalDomain=network_engine_domain  SubClassName=ps_output  LeftPortType=input  RightPortType=output  PseudoPeriodic=off  Frequencies=[]  Unit=1  AffineConversion=off
  z8 : nesl_utility/PS-Simulink Converter  PhysicalDomain=network_engine_domain  SubClassName=ps_output  LeftPortType=input  RightPortType=output  PseudoPeriodic=off  Frequencies=[]  Unit=1  AffineConversion=off
  Conn1 : PMIOPort  Port=1  Side=Left
  sensor_discrete_dz : Outport
  sensor_discrete_z : Outport  Port=2
  sensor_actual_z : Outport  Port=3
  wires:
  Kp10/1 -> Zero-Order Hold1/1, Transport Delay/1
  Discrete Derivative/1 -> sensor_discrete_dz/1
  Zero-Order Hold/1 -> sensor_discrete_z/1, Scope9/1, Discrete Derivative/1
  Zero-Order Hold1/1 -> Scope9/2
  Transport Delay/1 -> Zero-Order Hold/1
  z8/1 -> Kp10/1, sensor_actual_z/1
  Kp2/1 -> Kp1/1
  Product/1 -> Kp2/1
  Kp1/1 -> Scope1/1, " s_ps2"/1
  z1/1 -> Switch/1, Switch/2
  Switch/1 -> Scope1/2, Product/2, Product/1
  Constant/1 -> Switch/3
  connections:
  Rigid Transform2/RConn1 -- Universal Joint1/LConn1
  Rigid Transform3/RConn1 -- Link2/RConn1
  Rigid Transform2/LConn1 -- Conn1/RConn1
  World Frame1/RConn1 -- 6-DOF Joint1/LConn1
  z8/LConn1 -- 6-DOF Joint1/RConn2
  6-DOF Joint1/RConn1 -- Rigid Transform8/RConn1 -- SENSOR/RConn1
  Universal Joint1/RConn1 -- Link X+6/LConn1 -- Rigid Transform3/LConn1
  6-DOF Joint1/RConn3 -- z1/LConn1
  " s_ps2"/RConn1 -- 6-DOF Joint1/LConn2
  Rigid Transform8/LConn1 -- Link X+8/RConn1
  Link X+6/RConn1 -- Link X-2/LConn1
  Link X+1/RConn1 -- Link X-1/LConn1
  Link X+2/RConn1 -- Link X-4/LConn1
  Link X+5/RConn1 -- Link X-3/LConn1
  Link X+2/LConn1 -- Link X-1/RConn1
  Link X+3/RConn1 -- Link X-6/LConn1
  Link X+3/LConn1 -- Link X-3/RConn1
  Link X+4/LConn1 -- Link X-6/RConn1
  Link X+5/LConn1 -- Link X-4/RConn1
  Link X+1/LConn1 -- Link X-2/RConn1
  Link X+4/RConn1 -- Link X-5/LConn1
  Link X+7/LConn1 -- Link X-5/RConn1
  Link X+7/RConn1 -- Link X-7/LConn1
  Link X+8/LConn1 -- Link X-7/RConn1

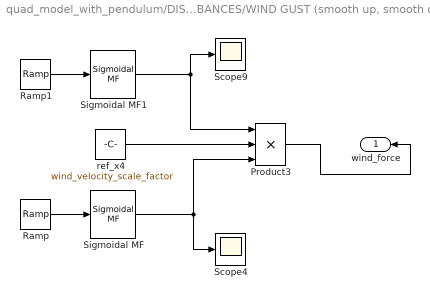
== system quad_model_with_pendulum/DISTURBANCES/WIND GUST (smooth up, smooth down)  ==
  Product3 : Product  Inputs=3
  Ramp : simulink/Sources/Ramp  slope=2  start=0  X0=-5
  Ramp1 : simulink/Sources/Ramp  slope=2  start=4  X0=-5
  Scope4 : Scope
  Scope9 : Scope
  Sigmoidal MF : fuzblock/Membership  Functions/Sigmoidal MF  a=1  c=0
  Sigmoidal MF1 : fuzblock/Membership  Functions/Sigmoidal MF  a=-1  c=0
  ref_x4 : Constant  Value=wind_velocity_scale_factor
  wind_force : Outport
  wires:
  Sigmoidal MF1/1 -> Product3/1, Scope9/1
  Ramp1/1 -> Sigmoidal MF1/1
  Ramp/1 -> Sigmoidal MF/1
  Sigmoidal MF/1 -> Product3/3, Scope4/1
  ref_x4/1 -> Product3/2
  Product3/1 -> wind_force/1
